simulink model "proyecto_con_componentes"  (R2017a)
settings: Solver=VariableStepAuto  StartTime=0.0  StopTime=5  RelTol=1e-3
undefined symbols (not defined in the file or in its folder): tf3
libraries: powerlib_meascontrol x1
settings Model: Creator=Gaby  LastModifiedBy=Gaby

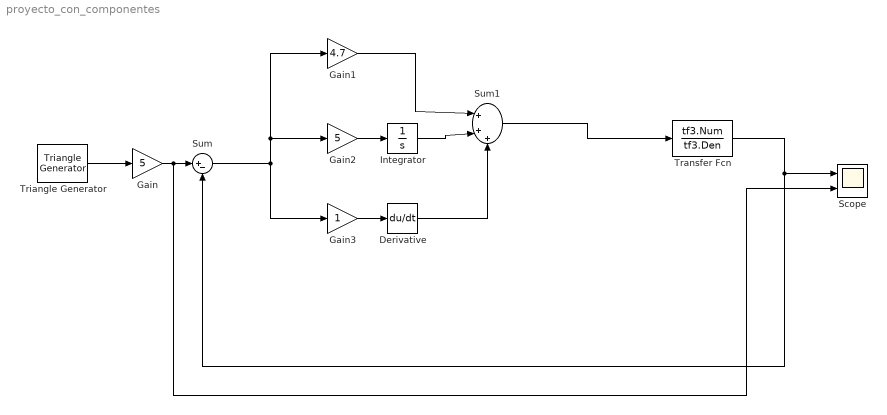
== system proyecto_con_componentes ==
  Derivative : Derivative
  Gain : Gain  Gain=5
  Gain1 : Gain  Gain=4.7
  Gain2 : Gain  Gain=5
  Gain3 : Gain
  Integrator : Integrator
  Scope : Scope  NumInputPorts=2
  Sum : Sum  Inputs=|+-
  Sum1 : Sum  Inputs=|+++
  Transfer Fcn : TransferFcn  Numerator=tf3.Num  Denominator=tf3.Den
  Triangle Generator : powerlib_meascontrol/Pulse & Signal Generators/Triangle Generator  Freq=0.5  Phase=90  Ts=0
  wires:
  Transfer Fcn/1 -> Sum/2, Scope/1
  Triangle Generator/1 -> Gain/1
  Gain/1 -> Scope/2, Sum/1
  Gain3/1 -> Derivative/1
  Gain2/1 -> Integrator/1
  Gain1/1 -> Sum1/1
  Integrator/1 -> Sum1/2
  Derivative/1 -> Sum1/3
  Sum/1 -> Gain3/1, Gain2/1, Gain1/1
  Sum1/1 -> Transfer Fcn/1
